simulink model "s9_template"  (R2023a)
settings: Solver=ode4  StartTime=0.0  StopTime=inf  FixedStep=P_sim_dt  RelTol=1e-3
InitFcn:
  | s6_data;
values from neighbouring files (symbols this model uses):
  a1total = 2.7    [mbc_teamchallenge_track.m]    (also in s6_data.m)
  a2total = 1.8    [mbc_teamchallenge_track.m]    (also in s6_data.m)
  breakslen = varargin{1}    [mbc_ppval.m]
  CarInputsCmdForward = uint8(1)    [p_mad_car.m]
  CarInputsCmdHalt = uint8(0)    [p_mad_car.m]
  CarInputsCmdReverse = uint8(2)    [p_mad_car.m]
  ManeuverTypePark = uint8(1)    [p_mad_car.m]
  ManeuverTypePathFollow = uint8(3)    [p_mad_car.m]
  P_cx_k = 1    [s6_data.m]
  P_p_Bf = 0.7    [p_mad_car.m]
  P_p_Br = 0.7    [p_mad_car.m]
  P_p_Cf = 2    [p_mad_car.m]
  P_p_Cr = 2    [p_mad_car.m]
  P_p_delta_max = 21.58/180*pi    (= 0.37664205258)    [p_mad_car.m]
  P_p_Df = 2    [p_mad_car.m]
  P_p_Dr = 2.5    [p_mad_car.m]
  P_p_Ef = -0.1    [p_mad_car.m]
  P_p_Er = -0.05    [p_mad_car.m]
  P_p_J = 192e-6    (= 0.000192)    [p_mad_car.m]
  P_p_k = 2.51    [p_mad_car.m]
  P_p_kr = 0.344014    [s6_data.m]
  P_p_l = abs(P_p_frontaxle_1 + P_p_rearaxle_1)    [p_mad_car.m]
  P_p_lf = P_p_frontaxle_1    (= 0.05)    [p_mad_car.m]
  P_p_lr = P_p_rearaxle_1    (= 0.049)    [p_mad_car.m]
  P_p_m = 132e-3    (= 0.132)    [p_mad_car.m]
  P_p_s1_start = 0.63    [s6_data.m]
  P_p_s2_start = 0.15    [s6_data.m]
  P_p_T = 316e-3    (= 0.316)    [p_mad_car.m]
  P_p_TA = 0.02    [s6_data.m]
  P_p_Ti = 0.246830    (= 0.24683)    [s6_data.m]
  P_p_Tt = P_p_uTt + P_p_output_Tt    (= 0.1)    [p_mad_car.m]
  P_p_Tw = 0.3    [s6_data.m]
  P_w_breakslen = uint32(length(path.points))    [s6_data.m]
  P_w_coefs = zeros(SPLINE.Elements(3).Dimensions)    [s6_data.m]
  P_w_points = zeros(SPLINE.Elements(2).Dimensions)    [s6_data.m]
  P_w_segments = uint32(zeros(SPLINE.Elements(4).Dimensions))    [s6_data.m]
  points = [ p.x + x ;      center1 + sign(t.xe) * r * cos(p.psi - pi/2 + sign(t.xe) * x / t.r) ;      center2 + sign(t.xe) * r * sin(p.psi - pi/2 + sign(t.xe) * x / t.r) ]    [mbc_circle_get_points.m]    (also in mbc_clothoid_get_points.m = [ p.x + x ;      s1;      s2]; mbc_spline_create.m = [ points(:, 1:end-1) [ points(1, end); points(2:3, 1) ] ]; mbc_straight_get_points.m = [ p.x + x ;      p.s1 + cpsi * x + (alpha - 0.5) * t.w * cos)
undefined symbols (not defined in the file or in its folder): coefs, DiscIntNeverNeededParam, periodic, segments
libraries: simulink x1, mad_lib_template x1
settings Model: Creator=hmekiedj  LastModifiedBy=aaron
settings DataIOCC: ReturnWorkspaceOutputs=off
settings OptimizationCC: BlockReduction=off  DefaultParameterBehavior=Inlined  BufferReuse=off
settings DebuggingCC: UnconnectedInputMsg=warning  UnconnectedOutputMsg=warning  UnconnectedLineMsg=warning  ArithmeticOperatorsInVariantConditions=warning
settings ModelReferenceCC: EnableRefExpFcnMdlSchedulingChecks=on
settings SFSimCC: SimUseLocalCustomCode=off  CustomCodeUndefinedFunction=UseInterfaceOnly
settings RTWCC: RTWUseLocalCustomCode=off  DLArmComputeVersion=19.05
settings CodeAppCC: StateflowObjectComments=on

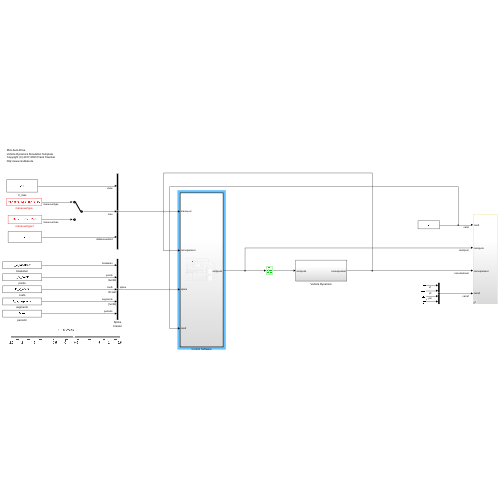
[thumbnail: Simulink's stored preview of the top-level diagram]
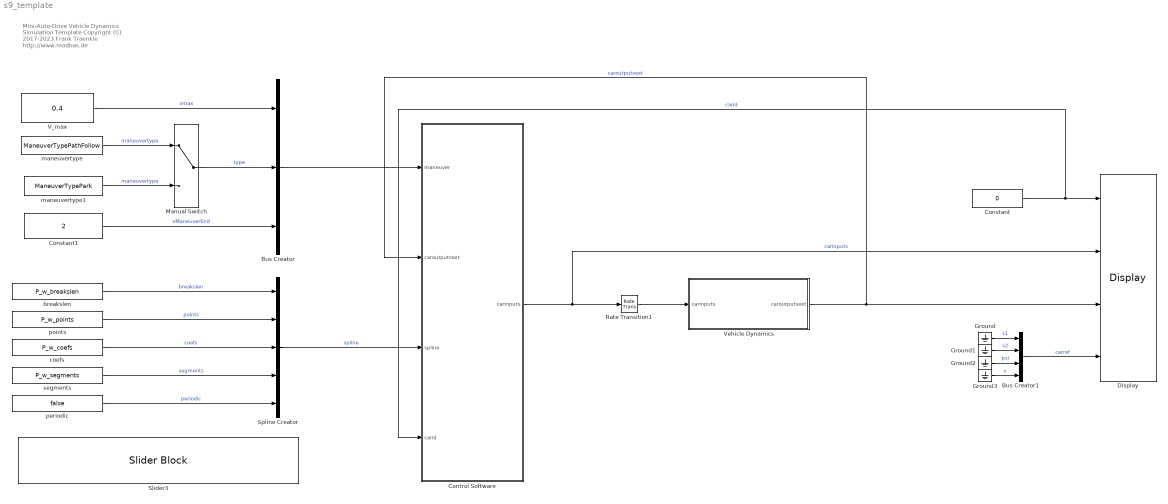
== system s9_template ==
  note: Mini-Auto-Drive
      | Vehicle Dynamics Simulation Template
      | Copyright (C) 2017-2023 Frank Traenkle
      | http://www.modbas.de
  Bus Creator : BusCreator  Inputs=3
  Bus Creator1 : BusCreator  Inputs=4
  Constant : Constant  Value=0
  Constant1 : Constant  Value=2
  Control Software : Subsystem  TreatAsAtomicUnit=on  SystemSampleTime=P_p_TA
  Display : mad_lib_template/Display  SystemSampleTime=-1  VariantActivationTime=update diagram  Latency=0  AutoFrameSizeCalculation=off
  Ground{,1..3} (4 alike) : Ground
  Manual Switch : ManualSwitch
  Rate Transition1 : RateTransition
  Slider3 : SliderBlock  ScaleMin=-2.50  ScaleMax=2.50  TickInterval=0.5
  Spline Creator : BusCreator  Inputs=breakslen,points,coefs,segments,periodic  OutDataTypeStr=Bus: SPLINE
  V_max : Constant  Value=0.4
  Vehicle Dynamics : Subsystem
  breakslen : Constant  Value=P_w_breakslen
  coefs : Constant  Value=P_w_coefs
  maneuvertype : Constant  Value=ManeuverTypePathFollow  SampleTime=-1
  maneuvertype1 : Constant  Value=ManeuverTypePark  SampleTime=-1
  periodic : Constant  Value=false
  points : Constant  Value=P_w_points
  segments : Constant  Value=P_w_segments
  wires:
  Bus Creator1/1 -> Display/4  "carref"
  Ground/1 -> Bus Creator1/1  "s1"
  Ground1/1 -> Bus Creator1/2  "s2"
  Ground2/1 -> Bus Creator1/3  "psi"
  Ground3/1 -> Bus Creator1/4  "v"
  Vehicle Dynamics/1(caroutputsext) -> Control Software/2(caroutputsext), Display/3  "caroutputsext"
  Rate Transition1/1 -> Vehicle Dynamics/1(carinputs)
  Control Software/1(carinputs) -> Display/2, Rate Transition1/1  "carinputs"
  Bus Creator/1 -> Control Software/1(maneuver)
  V_max/1 -> Bus Creator/1  "vmax"
  Manual Switch/1 -> Bus Creator/2  "type"
  maneuvertype/1 -> Manual Switch/1  "maneuvertype"
  maneuvertype1/1 -> Manual Switch/2  "maneuvertype"
  Constant1/1 -> Bus Creator/3  "xManeuverEnd"
  periodic/1 -> Spline Creator/5  "periodic"
  coefs/1 -> Spline Creator/3  "coefs"
  points/1 -> Spline Creator/2  "points"
  breakslen/1 -> Spline Creator/1  "breakslen"
  segments/1 -> Spline Creator/4  "segments"
  Spline Creator/1 -> Control Software/3(spline)  "spline"
  Constant/1 -> Display/1, Control Software/4(carid)  "carid"

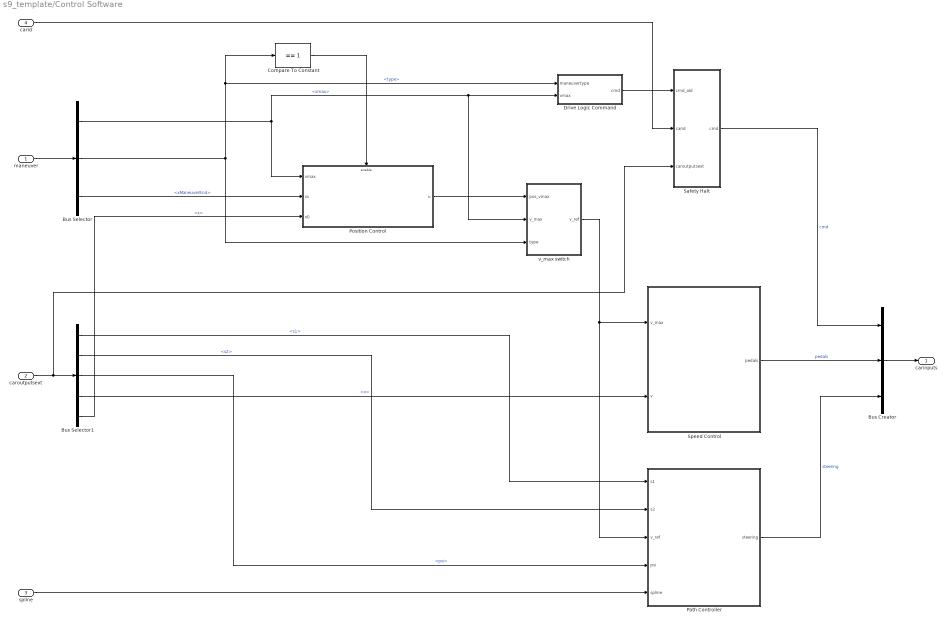
== system s9_template/Control Software ==
  maneuver : Inport
  caroutputsext : Inport  Port=2
  spline : Inport  Port=3
  carid : Inport  Port=4
  Bus Creator : BusCreator  Inputs=3
  Bus Selector : BusSelector  OutputSignals=vmax,type,xManeuverEnd
  Bus Selector1 : BusSelector  OutputSignals=s1,s2,psi,v,x
  Compare To Constant : simulink/Logic and Bit Operations/Compare To Constant  relop===  const=1  OutDataTypeStr=boolean
  Drive Logic Command : MATLAB Function  TreatAsAtomicUnit=on
  Path Controller : Subsystem
  Position Control : Subsystem  TreatAsAtomicUnit=on
  Safety Halt : MATLAB Function  TreatAsAtomicUnit=on
  Speed Control : Subsystem
  v_max switch : MATLAB Function  TreatAsAtomicUnit=on
  carinputs : Outport
  wires:
  caroutputsext/1 -> Bus Selector1/1, Safety Halt/3(caroutputsext)
  Position Control/1(u) -> v_max switch/1(pos_vmax)
  maneuver/1 -> Bus Selector/1
  Bus Selector/1 -> Position Control/1(vmax), v_max switch/2(v_max), Drive Logic Command/2(vmax)  "<vmax>"
  Bus Selector1/5 -> Position Control/3(x0)  "<x>"
  Bus Selector/2 -> v_max switch/3(type), Compare To Constant/1, Drive Logic Command/1(maneuvertype)  "<type>"
  Compare To Constant/1 -> Position Control/Enable
  Bus Creator/1 -> carinputs/1
  Bus Selector/3 -> Position Control/2(xs)  "<xManeuverEnd>"
  Bus Selector1/1 -> Path Controller/1(s1)  "<s1>"
  Bus Selector1/2 -> Path Controller/2(s2)  "<s2>"
  Bus Selector1/3 -> Path Controller/4(psi)  "<psi>"
  v_max switch/1(v_ref) -> Path Controller/3(v_ref), Speed Control/1(v_max)
  Drive Logic Command/1(cmd) -> Safety Halt/1(cmd_old)
  Path Controller/1(steering) -> Bus Creator/3  "steering"
  spline/1 -> Path Controller/5(spline)
  Bus Selector1/4 -> Speed Control/2(v)  "<v>"
  Speed Control/1(pedals) -> Bus Creator/2  "pedals"
  Safety Halt/1(cmd) -> Bus Creator/1  "cmd"
  carid/1 -> Safety Halt/2(carid)

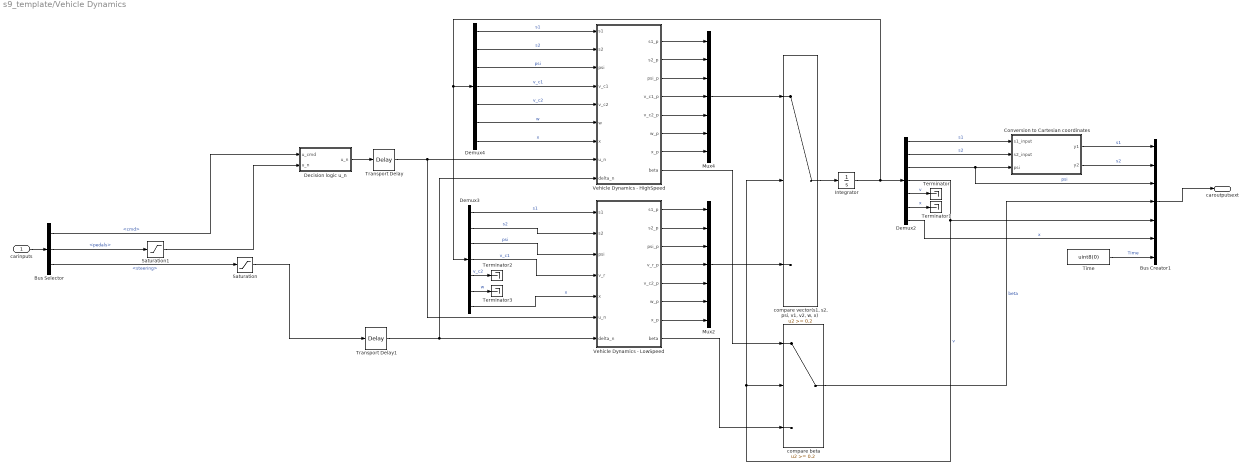
== system s9_template/Vehicle Dynamics ==
  carinputs : Inport
  Bus Creator1 : BusCreator  Inputs=7  OutDataTypeStr=Bus: CAROUTPUTSEXT
  Bus Selector : BusSelector  OutputSignals=cmd,pedals,steering
  Conversion to Cartesian coordinates : MATLAB Function  TreatAsAtomicUnit=on
  Decision logic u_n : MATLAB Function  TreatAsAtomicUnit=on
  Demux2 : Demux  Outputs=7
  Demux3 : Demux  Outputs=7
  Demux4 : Demux  Outputs=7
  Integrator : Integrator  InitialCondition=[P_p_s1_start; P_p_s2_start; 0; 0; 0; 0; 0]
  Mux2 : Mux  Inputs=7
  Mux4 : Mux  Inputs=7
  Saturation : Saturate  UpperLimit=1  LowerLimit=-1
  Saturation1 : Saturate  UpperLimit=1  LowerLimit=-1
  Terminator{,1..3} (4 alike) : Terminator
  Time : Constant  Value=uint8(0)
  Transport Delay : TransportDelay  DelayTime=P_p_Tt
  Transport Delay1 : TransportDelay  DelayTime=P_p_Tt
  Vehicle Dynamics - HighSpeed : Subsystem
  Vehicle Dynamics - LowSpeed : Subsystem
  compare beta : Switch  Threshold=0.2  SaturateOnIntegerOverflow=off  InputSameDT=off
  "compare vector(s1, s2, psi, v1, v2, w, x)" : Switch  Threshold=0.2  SaturateOnIntegerOverflow=off  InputSameDT=off
  caroutputsext : Outport  VectorParamsAs1DForOutWhenUnconnected=off
  wires:
  carinputs/1 -> Bus Selector/1
  Bus Selector/2 -> Saturation1/1  "<pedals>"
  Bus Selector/3 -> Saturation/1  "<steering>"
  Demux2/3 -> Conversion to Cartesian coordinates/3(psi), Bus Creator1/3  "psi"
  Bus Creator1/1 -> caroutputsext/1
  Demux2/7 -> Bus Creator1/6  "x"
  Demux2/2 -> Conversion to Cartesian coordinates/2(s2_input)  "s2"
  Demux2/1 -> Conversion to Cartesian coordinates/1(s1_input)  "s1"
  Bus Selector/1 -> Decision logic u_n/1(u_cmd)  "<cmd>"
  Saturation1/1 -> Decision logic u_n/2("u_n ")
  Saturation/1 -> Transport Delay1/1
  Vehicle Dynamics - HighSpeed/1(s1_p) -> Mux4/1
  Vehicle Dynamics - HighSpeed/2(s2_p) -> Mux4/2
  Vehicle Dynamics - HighSpeed/3(psi_p) -> Mux4/3
  Vehicle Dynamics - HighSpeed/4(v_c1_p) -> Mux4/4
  Vehicle Dynamics - HighSpeed/5(v_c2_p) -> Mux4/5
  Vehicle Dynamics - HighSpeed/6(w_p) -> Mux4/6
  Vehicle Dynamics - HighSpeed/7(x_p) -> Mux4/7
  Vehicle Dynamics - LowSpeed/1(s1_p) -> Mux2/1
  Vehicle Dynamics - LowSpeed/2(s2_p) -> Mux2/2
  Vehicle Dynamics - LowSpeed/3(psi_p) -> Mux2/3
  Vehicle Dynamics - LowSpeed/4(v_r_p) -> Mux2/4
  Vehicle Dynamics - LowSpeed/5(v_c2_p) -> Mux2/5
  Vehicle Dynamics - LowSpeed/6(w_p) -> Mux2/6
  Vehicle Dynamics - LowSpeed/7(x_p) -> Mux2/7
  Mux4/1 -> "compare vector(s1, s2, psi, v1, v2, w, x)"/1
  "compare vector(s1, s2, psi, v1, v2, w, x)"/1 -> Integrator/1
  Integrator/1 -> Demux2/1, Demux4/1, Demux3/1
  Demux2/4 -> "compare vector(s1, s2, psi, v1, v2, w, x)"/2, compare beta/2, Bus Creator1/5  "v"
  Demux3/1 -> Vehicle Dynamics - LowSpeed/1(s1)  "s1"
  Demux3/2 -> Vehicle Dynamics - LowSpeed/2(s2)  "s2"
  Demux3/3 -> Vehicle Dynamics - LowSpeed/3(psi)  "psi"
  Demux3/4 -> Vehicle Dynamics - LowSpeed/4(v_r)  "v_c1"
  Demux3/7 -> Vehicle Dynamics - LowSpeed/5(x)  "x"
  Demux4/1 -> Vehicle Dynamics - HighSpeed/1(s1)  "s1"
  Demux4/2 -> Vehicle Dynamics - HighSpeed/2(s2)  "s2"
  Demux4/3 -> Vehicle Dynamics - HighSpeed/3(psi)  "psi"
  Demux4/4 -> Vehicle Dynamics - HighSpeed/4(v_c1)  "v_c1"
  Demux4/5 -> Vehicle Dynamics - HighSpeed/5(v_c2)  "v_c2"
  Demux4/6 -> Vehicle Dynamics - HighSpeed/6(w)  "w"
  Demux4/7 -> Vehicle Dynamics - HighSpeed/7(x)  "x"
  Transport Delay/1 -> Vehicle Dynamics - LowSpeed/6(u_n), Vehicle Dynamics - HighSpeed/8(u_n)
  Transport Delay1/1 -> Vehicle Dynamics - LowSpeed/7(delta_n), Vehicle Dynamics - HighSpeed/9(delta_n)
  Vehicle Dynamics - LowSpeed/8(beta) -> compare beta/3
  Vehicle Dynamics - HighSpeed/8(beta) -> compare beta/1
  compare beta/1 -> Bus Creator1/4  "beta"
  Conversion to Cartesian coordinates/1(y1) -> Bus Creator1/1  "s1"
  Conversion to Cartesian coordinates/2(y2) -> Bus Creator1/2  "s2"
  Demux2/5 -> Terminator/1  "v"
  Demux2/6 -> Terminator1/1  "x"
  Decision logic u_n/1(u_n) -> Transport Delay/1
  Demux3/5 -> Terminator2/1  "v_c2"
  Demux3/6 -> Terminator3/1  "w"
  Mux2/1 -> "compare vector(s1, s2, psi, v1, v2, w, x)"/3
  Time/1 -> Bus Creator1/7  "Time"

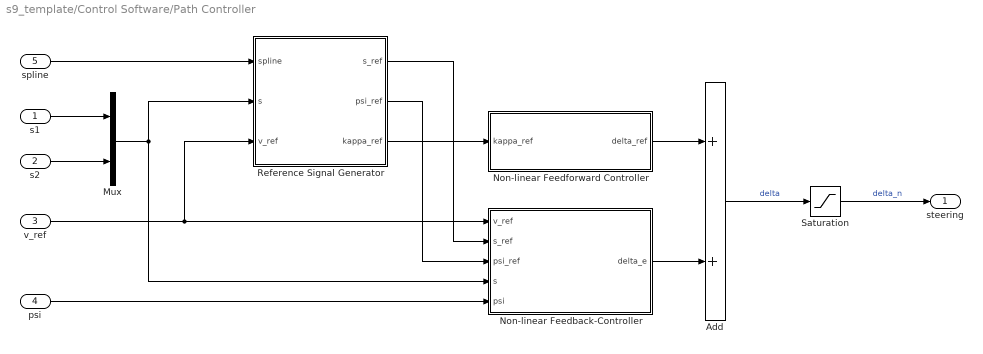
== system s9_template/Control Software/Path Controller ==
  s1 : Inport
  s2 : Inport  Port=2
  v_ref : Inport  Port=3
  psi : Inport  Port=4
  spline : Inport  Port=5
  Add : Sum
  Mux : Mux  Inputs=2
  Non-linear Feedback-Controller : MATLAB Function  TreatAsAtomicUnit=on
  Non-linear Feedforward Controller : MATLAB Function  TreatAsAtomicUnit=on
  Reference Signal Generator : MATLAB Function  TreatAsAtomicUnit=on
  Saturation : Saturate  UpperLimit=1  LowerLimit=-1
  steering : Outport
  wires:
  spline/1 -> Reference Signal Generator/1(spline)
  s1/1 -> Mux/1
  s2/1 -> Mux/2
  v_ref/1 -> Reference Signal Generator/3(v_ref), Non-linear Feedback-Controller/1(v_ref)
  Reference Signal Generator/3(kappa_ref) -> Non-linear Feedforward Controller/1(kappa_ref)
  Reference Signal Generator/2(psi_ref) -> Non-linear Feedback-Controller/3(psi_ref)
  Reference Signal Generator/1(s_ref) -> Non-linear Feedback-Controller/2(s_ref)
  Non-linear Feedforward Controller/1(delta_ref) -> Add/1
  Non-linear Feedback-Controller/1(delta_e) -> Add/2
  Add/1 -> Saturation/1  "delta"
  Saturation/1 -> steering/1  "delta_n"
  Mux/1 -> Reference Signal Generator/2(s), Non-linear Feedback-Controller/4(s)
  psi/1 -> Non-linear Feedback-Controller/5(psi)

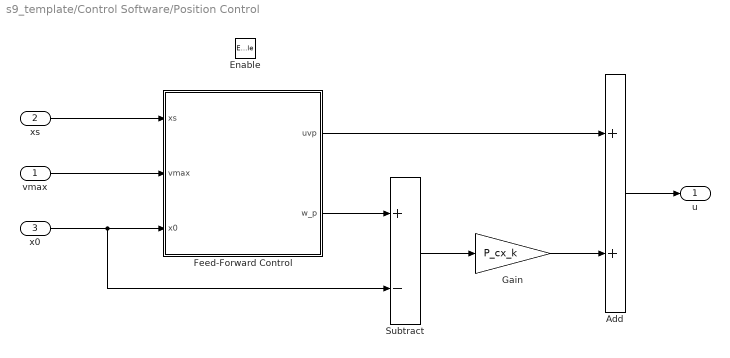
== system s9_template/Control Software/Position Control ==
  vmax : Inport
  xs : Inport  Port=2
  x0 : Inport  Port=3
  Enable : EnablePort
  Add : Sum
  Feed-Forward Control : Subsystem
  Gain : Gain  Gain=P_cx_k
  Subtract : Sum  Inputs=+-
  u : Outport
  wires:
  xs/1 -> Feed-Forward Control/1(xs)
  Feed-Forward Control/2(w_p) -> Subtract/1
  Subtract/1 -> Gain/1
  Feed-Forward Control/1(uvp) -> Add/1
  vmax/1 -> Feed-Forward Control/2(vmax)
  Gain/1 -> Add/2
  Add/1 -> u/1
  x0/1 -> Subtract/2, Feed-Forward Control/3(x0)

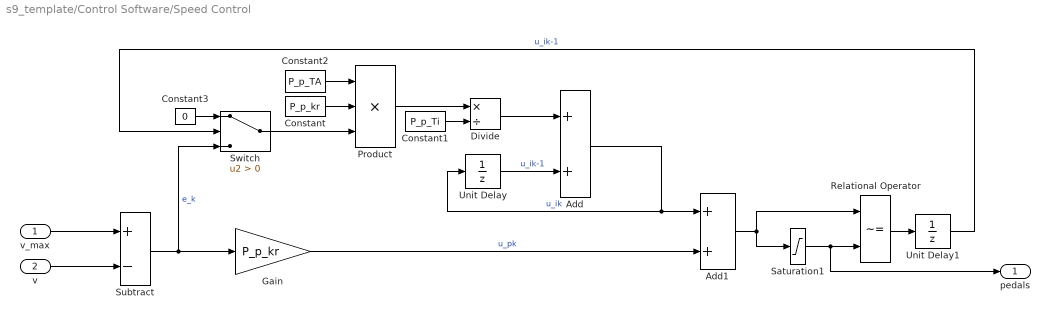
== system s9_template/Control Software/Speed Control ==
  v_max : Inport
  v : Inport  Port=2
  Add : Sum
  Add1 : Sum
  Constant : Constant  Value=P_p_kr
  Constant1 : Constant  Value=P_p_Ti  VectorParams1D=off
  Constant2 : Constant  Value=P_p_TA  VectorParams1D=off
  Constant3 : Constant  Value=0
  Divide : Product  Inputs=*/
  Gain : Gain  Gain=P_p_kr
  Product : Product  Inputs=3
  Relational Operator : RelationalOperator  Operator=~=  OutDataTypeStr=boolean  RndMeth=Simplest  InputSameDT=off
  Saturation1 : Saturate  UpperLimit=1  LowerLimit=-1
  Subtract : Sum  Inputs=+-
  Switch : Switch  Criteria=u2 > Threshold  SaturateOnIntegerOverflow=off  InputSameDT=off
  Unit Delay : UnitDelay  SampleTime=P_p_TA  HasFrameUpgradeWarning=on
  Unit Delay1 : UnitDelay  SampleTime=P_p_TA  HasFrameUpgradeWarning=on
  pedals : Outport
  wires:
  Constant3/1 -> Switch/1
  Relational Operator/1 -> Unit Delay1/1
  Divide/1 -> Add/1
  Subtract/1 -> Gain/1, Switch/3  "e_k"
  Constant2/1 -> Product/1
  Saturation1/1 -> Relational Operator/2, pedals/1
  Switch/1 -> Product/3
  Constant/1 -> Product/2
  Constant1/1 -> Divide/2
  Product/1 -> Divide/1
  Unit Delay1/1 -> Switch/2  "u_ik-1"
  Gain/1 -> Add1/2  "u_pk"
  Unit Delay/1 -> Add/2  "u_ik-1"
  Add/1 -> Add1/1, Unit Delay/1  "u_ik"
  Add1/1 -> Relational Operator/1, Saturation1/1
  v_max/1 -> Subtract/1
  v/1 -> Subtract/2

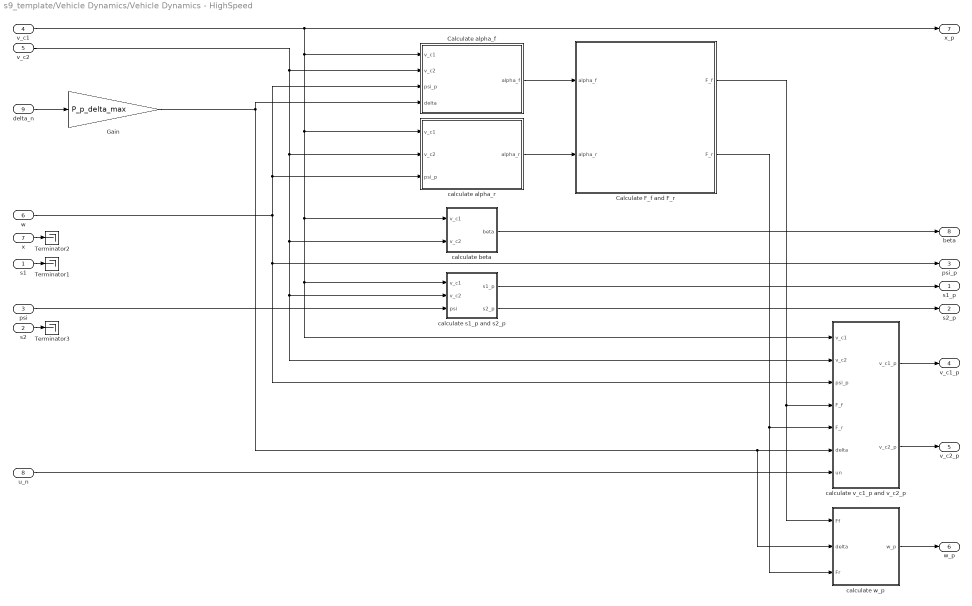
== system s9_template/Vehicle Dynamics/Vehicle Dynamics - HighSpeed ==
  s1 : Inport
  s2 : Inport  Port=2
  psi : Inport  Port=3
  v_c1 : Inport  Port=4
  v_c2 : Inport  Port=5
  w : Inport  Port=6
  x : Inport  Port=7
  u_n : Inport  Port=8
  delta_n : Inport  Port=9
  Calculate F_f and F_r : MATLAB Function  TreatAsAtomicUnit=on
  Calculate alpha_f : MATLAB Function  TreatAsAtomicUnit=on
  Gain : Gain  Gain=P_p_delta_max
  Terminator1 : Terminator
  Terminator2 : Terminator
  Terminator3 : Terminator
  calculate alpha_r : MATLAB Function  TreatAsAtomicUnit=on
  calculate beta : MATLAB Function  TreatAsAtomicUnit=on
  calculate s1_p and s2_p : MATLAB Function  TreatAsAtomicUnit=on
  calculate v_c1_p and v_c2_p : MATLAB Function  TreatAsAtomicUnit=on
  calculate w_p : MATLAB Function  TreatAsAtomicUnit=on
  s1_p : Outport  VectorParamsAs1DForOutWhenUnconnected=off
  s2_p : Outport  Port=2  VectorParamsAs1DForOutWhenUnconnected=off
  psi_p : Outport  Port=3  VectorParamsAs1DForOutWhenUnconnected=off
  v_c1_p : Outport  Port=4  VectorParamsAs1DForOutWhenUnconnected=off
  v_c2_p : Outport  Port=5  VectorParamsAs1DForOutWhenUnconnected=off
  w_p : Outport  Port=6  VectorParamsAs1DForOutWhenUnconnected=off
  x_p : Outport  Port=7  VectorParamsAs1DForOutWhenUnconnected=off
  beta : Outport  Port=8  VectorParamsAs1DForOutWhenUnconnected=off
  wires:
  delta_n/1 -> Gain/1
  Calculate alpha_f/1(alpha_f) -> Calculate F_f and F_r/1(alpha_f)
  calculate alpha_r/1(alpha_r) -> Calculate F_f and F_r/2(alpha_r)
  calculate beta/1(beta) -> beta/1
  calculate s1_p and s2_p/1(s1_p) -> s1_p/1
  calculate s1_p and s2_p/2(s2_p) -> s2_p/1
  Gain/1 -> calculate v_c1_p and v_c2_p/6(delta), calculate w_p/2(delta), Calculate alpha_f/4(delta)
  w/1 -> psi_p/1, calculate v_c1_p and v_c2_p/3(psi_p), calculate alpha_r/3(psi_p), Calculate alpha_f/3(psi_p)
  u_n/1 -> calculate v_c1_p and v_c2_p/7(un)
  Calculate F_f and F_r/2(F_r) -> calculate w_p/3(Fr), calculate v_c1_p and v_c2_p/5(F_r)
  Calculate F_f and F_r/1(F_f) -> calculate w_p/1(Ff), calculate v_c1_p and v_c2_p/4(F_f)
  calculate v_c1_p and v_c2_p/1(v_c1_p) -> v_c1_p/1
  calculate v_c1_p and v_c2_p/2(v_c2_p) -> v_c2_p/1
  v_c1/1 -> calculate v_c1_p and v_c2_p/1(v_c1), calculate s1_p and s2_p/1(v_c1), calculate beta/1(v_c1), calculate alpha_r/1(v_c1), Calculate alpha_f/1(v_c1), x_p/1
  v_c2/1 -> calculate v_c1_p and v_c2_p/2(v_c2), calculate s1_p and s2_p/2(v_c2), calculate beta/2(v_c2), calculate alpha_r/2(v_c2), Calculate alpha_f/2(v_c2)
  calculate w_p/1(w_p) -> w_p/1
  psi/1 -> calculate s1_p and s2_p/3(psi)
  x/1 -> Terminator2/1
  s1/1 -> Terminator1/1
  s2/1 -> Terminator3/1

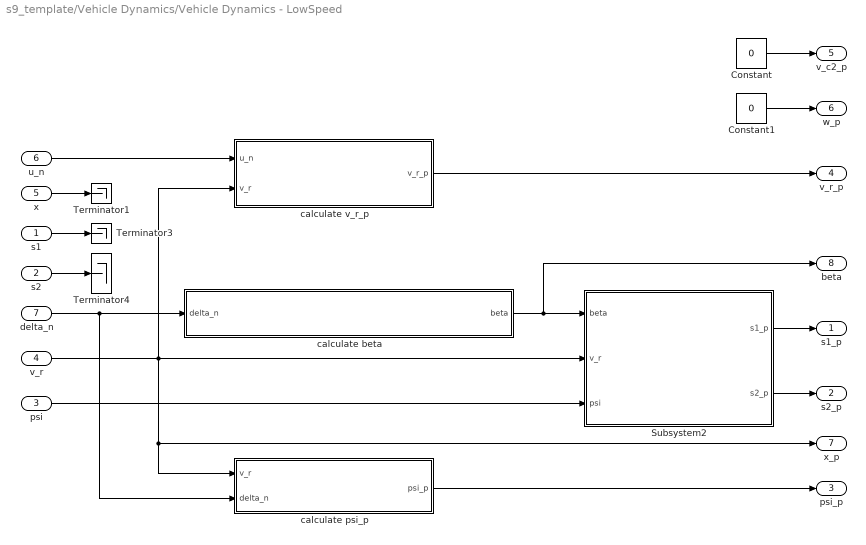
== system s9_template/Vehicle Dynamics/Vehicle Dynamics - LowSpeed ==
  s1 : Inport
  s2 : Inport  Port=2
  psi : Inport  Port=3
  v_r : Inport  Port=4
  x : Inport  Port=5
  u_n : Inport  Port=6
  delta_n : Inport  Port=7
  Constant : Constant  Value=0
  Constant1 : Constant  Value=0
  Subsystem2 : Subsystem
  Terminator1 : Terminator
  Terminator3 : Terminator
  Terminator4 : Terminator
  calculate beta : Subsystem
  calculate psi_p : Subsystem
  calculate v_r_p : Subsystem
  s1_p : Outport  VectorParamsAs1DForOutWhenUnconnected=off
  s2_p : Outport  Port=2  VectorParamsAs1DForOutWhenUnconnected=off
  psi_p : Outport  Port=3  VectorParamsAs1DForOutWhenUnconnected=off
  v_r_p : Outport  Port=4  VectorParamsAs1DForOutWhenUnconnected=off
  v_c2_p : Outport  Port=5  VectorParamsAs1DForOutWhenUnconnected=off
  w_p : Outport  Port=6  VectorParamsAs1DForOutWhenUnconnected=off
  x_p : Outport  Port=7  VectorParamsAs1DForOutWhenUnconnected=off
  beta : Outport  Port=8  VectorParamsAs1DForOutWhenUnconnected=off
  wires:
  u_n/1 -> calculate v_r_p/1(u_n)
  calculate v_r_p/1(v_r_p) -> v_r_p/1
  v_r/1 -> calculate psi_p/1(v_r), x_p/1, Subsystem2/2(v_r), calculate v_r_p/2(v_r)
  delta_n/1 -> calculate psi_p/2(delta_n), calculate beta/1(delta_n)
  Subsystem2/1(s1_p) -> s1_p/1
  psi/1 -> Subsystem2/3(psi)
  calculate beta/1(beta) -> Subsystem2/1(beta), beta/1
  Subsystem2/2(s2_p) -> s2_p/1
  calculate psi_p/1(psi_p) -> psi_p/1
  x/1 -> Terminator1/1
  s1/1 -> Terminator3/1
  s2/1 -> Terminator4/1
  Constant/1 -> v_c2_p/1
  Constant1/1 -> w_p/1

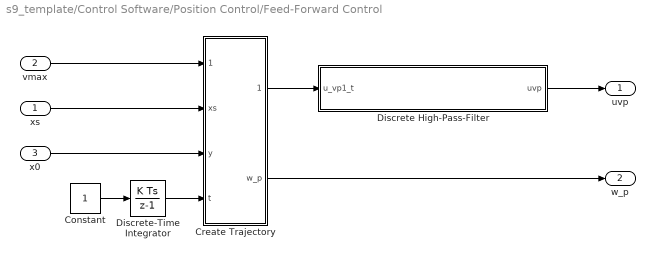
== system s9_template/Control Software/Position Control/Feed-Forward Control ==
  xs : Inport
  vmax : Inport  Port=2
  x0 : Inport  Port=3
  Constant : Constant
  "Create Trajectory " : MATLAB Function  TreatAsAtomicUnit=on
  Discrete High-Pass-Filter : Subsystem  TreatAsAtomicUnit=on
  Discrete-Time Integrator : DiscreteIntegrator  SampleTime=-1  ICPrevOutput=DiscIntNeverNeededParam  ICPrevScaledInput=DiscIntNeverNeededParam
  uvp : Outport
  w_p : Outport  Port=2
  wires:
  x0/1 -> "Create Trajectory "/3(y)
  vmax/1 -> "Create Trajectory "/1(vmax)
  xs/1 -> "Create Trajectory "/2(xs)
  "Create Trajectory "/2(w_p) -> w_p/1
  "Create Trajectory "/1(u_vp1_t) -> Discrete High-Pass-Filter/1(u_vp1_t)
  Constant/1 -> Discrete-Time Integrator/1
  Discrete-Time Integrator/1 -> "Create Trajectory "/4(t)
  Discrete High-Pass-Filter/1(uvp) -> uvp/1

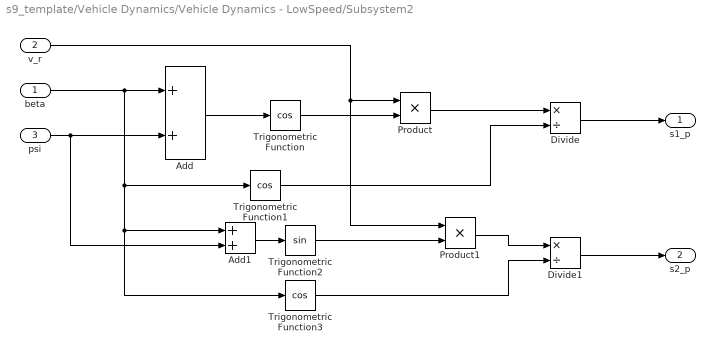
== system s9_template/Vehicle Dynamics/Vehicle Dynamics - LowSpeed/Subsystem2 ==
  beta : Inport
  v_r : Inport  Port=2
  psi : Inport  Port=3
  Add : Sum
  Add1 : Sum
  Divide : Product  Inputs=*/
  Divide1 : Product  Inputs=*/
  Product : Product
  Product1 : Product
  Trigonometric Function : Trigonometry  Operator=cos
  Trigonometric Function1 : Trigonometry  Operator=cos
  Trigonometric Function2 : Trigonometry
  Trigonometric Function3 : Trigonometry  Operator=cos
  s1_p : Outport  VectorParamsAs1DForOutWhenUnconnected=off
  s2_p : Outport  Port=2  VectorParamsAs1DForOutWhenUnconnected=off
  wires:
  Add/1 -> Trigonometric Function/1
  Trigonometric Function/1 -> Product/2
  Product/1 -> Divide/1
  Trigonometric Function1/1 -> Divide/2
  Divide/1 -> s1_p/1
  psi/1 -> Add1/2, Add/2
  beta/1 -> Trigonometric Function1/1, Trigonometric Function3/1, Add1/1, Add/1
  Trigonometric Function2/1 -> Product1/2
  Divide1/1 -> s2_p/1
  v_r/1 -> Product1/1, Product/1
  Product1/1 -> Divide1/1
  Add1/1 -> Trigonometric Function2/1
  Trigonometric Function3/1 -> Divide1/2

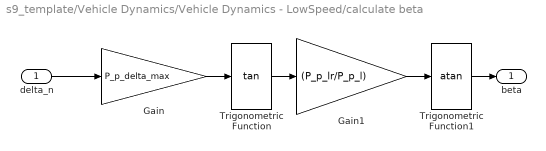
== system s9_template/Vehicle Dynamics/Vehicle Dynamics - LowSpeed/calculate beta ==
  delta_n : Inport
  Gain : Gain  Gain=P_p_delta_max
  Gain1 : Gain  Gain=(P_p_lr/P_p_l)
  Trigonometric Function : Trigonometry  Operator=tan
  Trigonometric Function1 : Trigonometry  Operator=atan
  beta : Outport  VectorParamsAs1DForOutWhenUnconnected=off
  wires:
  delta_n/1 -> Gain/1
  Gain/1 -> Trigonometric Function/1
  Trigonometric Function/1 -> Gain1/1
  Gain1/1 -> Trigonometric Function1/1
  Trigonometric Function1/1 -> beta/1

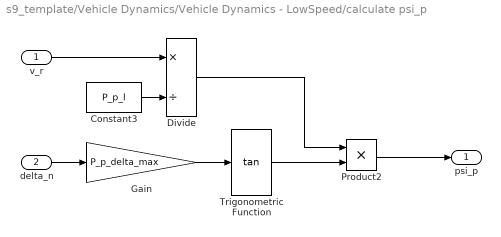
== system s9_template/Vehicle Dynamics/Vehicle Dynamics - LowSpeed/calculate psi_p ==
  v_r : Inport
  delta_n : Inport  Port=2
  Constant3 : Constant  Value=P_p_l
  Divide : Product  Inputs=*/
  Gain : Gain  Gain=P_p_delta_max
  Product2 : Product
  Trigonometric Function : Trigonometry  Operator=tan
  psi_p : Outport  VectorParamsAs1DForOutWhenUnconnected=off
  wires:
  delta_n/1 -> Gain/1
  Gain/1 -> Trigonometric Function/1
  Product2/1 -> psi_p/1
  v_r/1 -> Divide/1
  Constant3/1 -> Divide/2
  Trigonometric Function/1 -> Product2/2
  Divide/1 -> Product2/1

== system s9_template/Vehicle Dynamics/Vehicle Dynamics - LowSpeed/calculate v_r_p ==
  u_n : Inport
  v_r : Inport  Port=2
  Add : Sum  Inputs=-+
  Gain : Gain  Gain=(1/P_p_T)
  Gain1 : Gain  Gain=(P_p_k/P_p_T)
  v_r_p : Outport  VectorParamsAs1DForOutWhenUnconnected=off
  wires:
  Gain/1 -> Add/1
  Add/1 -> v_r_p/1
  v_r/1 -> Gain/1
  u_n/1 -> Gain1/1
  Gain1/1 -> Add/2

== system s9_template/Control Software/Position Control/Feed-Forward Control/Discrete High-Pass-Filter ==
  u_vp1_t : Inport
  Discrete High-Pass-Filter : DiscreteTransferFcn  Numerator=[2, -2]  Denominator=[(2*P_p_Ti+P_p_T) (P_p_T-2*P_p_Ti)]
  uvp : Outport
  wires:
  Discrete High-Pass-Filter/1 -> uvp/1
  u_vp1_t/1 -> Discrete High-Pass-Filter/1

== matlab function s9_template/Vehicle Dynamics/Vehicle Dynamics - HighSpeed/calculate v_c1_p and v_c2_p ==
  data: v_c1 input; v_c1_p output; v_c2 input; psi_p input; v_c2_p output; F_f input; F_r input; delta input; un input; P_p_m parameter; P_p_T parameter; P_p_k parameter
function [v_c1_p, v_c2_p] = fcn(v_c1, v_c2, psi_p, F_f, F_r, delta, un, P_p_m, P_p_T, P_p_k)
    % Function: fcn
    % Description: Calculates the updated longitudinal and lateral velocity components 
    %              of a vehicle based on various dynamic parameters and forces.
    %
    % Inputs:
    %   v_c1 - Initial longitudinal velocity component.
    %   v_c2 - Initial lateral velocity component.
    %   psi_p - Yaw rate of the vehicle.
    %   F_f - Tire force at the front of the vehicle.
    %   F_r - Tire force at the rear of the vehicle.
    %   delta - Steering angle.
    %   un - Motor control signal.
    %   P_p_m - Mass of the vehicle.
    %   P_p_T - Time constant related to the vehicle dynamics.
    %   P_p_k - Constant related to the motor control effectiveness.
    %
    % Outputs:
    %   v_c1_p - Updated longitudinal velocity component.
    %   v_c2_p - Updated lateral velocity component.
    %
    % The function calculates the new velocity components considering the external forces,
    % vehicle's yaw rate, steering angle, motor control signal, and various vehicle parameters.
    % These calculations are essential for understanding the vehicle's dynamic behavior under
    % different control inputs and conditions.
    
    % Calculating the updated velocity components
    v_c1_p = double((1 / P_p_m) * (-F_f * sin(delta) + (P_p_m * v_c2 * psi_p)) - (1 / P_p_T * v_c1) + ((P_p_k / P_p_T) * un));
    v_c2_p = double((1 / P_p_m) * (F_f * cos(delta) + F_r - (P_p_m * v_c1 * psi_p)));
end

== matlab function s9_template/Vehicle Dynamics/Vehicle Dynamics - HighSpeed/calculate w_p ==
  data: w_p output; Ff input; delta input; Fr input; P_p_J parameter; P_p_lf parameter; P_p_lr parameter
function w_p = fcn(Ff, delta, Fr, P_p_J, P_p_lf, P_p_lr)
    % Function: fcn
    % Description: Calculates the yaw rate change 'w_p' of a vehicle.
    %
    % Inputs:
    %   Ff - Front tire force.
    %   delta - Steering angle.
    %   Fr - Rear tire force.
    %   P_p_J - Moment of inertia of the vehicle about the yaw axis.
    %   P_p_lf - Distance from the center of gravity (COG) to the front axle.
    %   P_p_lr - Distance from the COG to the rear axle.
    %
    % Output:
    %   w_p - Calculated change in yaw rate.
    %
    % The function computes the change in the vehicle's yaw rate based on the forces 
    % acting on the front and rear tires, the steering angle, the vehicle's moment of 
    % inertia, and the distances from the COG to the front and rear axles. This calculation 
    % is crucial for understanding the vehicle's dynamic response to steering inputs.
    
    % Calculation of the yaw rate change 'w_p'
    w_p = 1 / P_p_J * (Ff * P_p_lf * cos(delta) - Fr * P_p_lr);
end

== matlab function s9_template/Control Software/Drive Logic Command ==
  data: maneuvertype input; vmax input; cmd output
function cmd = fcn(maneuvertype, vmax)
    % Function: fcn
    % Description: Determines the appropriate command for vehicle maneuver based on the 
    %              maneuver type and maximum velocity.
    %
    % Inputs:
    %   maneuvertype - Numeric value indicating the type of maneuver.
    %   vmax - Maximum velocity 
    %   CarInputsCmdReverse - Command for reversing the vehicle.
    %   CarInputsCmdForward - Command for moving the vehicle forward.
    %   CarInputsCmdSlow - Command for slowing down the vehicle.
    %
    % Output:
    %   cmd - The calculated command for the vehicle maneuver.
    %
    % The function sets the command for a vehicle maneuver based on the maneuver type and 
    % maximum velocity. If the maneuver type is 1, it sets the command to slow down. Otherwise, 
    % it chooses between moving forward or reversing based on the maximum velocity.

    % Setting the initial command to forward    
    % Logic to determine the command based on maneuver type and maximum velocity
    % if maneuvertype == 1
    %     cmd = CarInputsCmdSlow;
    % else
    %     if vmax >= 0
    %         cmd = CarInputsCmdForward;
    %     elseif vmax < 0
    %         cmd = CarInputsCmdReverse;
    %     end 
    % end
    cmd = 1;   % "CarInputsCmdForward"
      switch maneuvertype
        case 0      % CarInputsCmdHalt
            cmd = 0;
        case 1  % CarInputsCmdForward 
            if (vmax < 0)
                cmd = 0;
            end
        case 2  % CarInputsCmdReverse 
            if (vmax > 0)
                cmd = 0;
            end
     end
end

== matlab function s9_template/Control Software/Path Controller/Reference Signal Generator ==
  data: spline input; s_ref output; s input size=2; v_ref input size=1; psi_ref output; kappa_ref output; P_p_Tt parameter
function [s_ref, psi_ref, kappa_ref] = E_ref(spline, s, v_ref, P_p_Tt)
    % Function: E_ref
    % Description: Calculates reference values for position, orientation, and curvature
    %              based on a given spline, position, and velocity.
    %
    % Inputs:
    %   spline - Spline structure containing points, coefficients, lengths, and periodicity.
    %   s - Current position along the spline.
    %   v_ref - Reference velocity.
    %   P_p_Tt - Dead time affecting the response.
    %
    % Outputs:
    %   s_ref - Reference position in terms of x and y coordinates.
    %   psi_ref - Reference orientation (yaw angle).
    %   kappa_ref - Reference curvature.
    %
    % The function uses the spline data along with the current position and reference velocity
    % to determine the reference position (s_ref), orientation (psi_ref), and curvature (kappa_ref).
    % These are crucial for path following and trajectory planning in vehicle dynamics.
    %

    % Extracting spline components
    points = spline.points;
    coefs = spline.coefs;
    breakslen = spline.breakslen;
    periodic = spline.periodic;
    
    % Calculating reference values using spline data
    [w, widx] = mbc_spline_get_reference(s, breakslen, points, coefs, periodic, v_ref, P_p_Tt);
    
    % Assigning the calculated reference values
    psi_ref = w(2);
    kappa_ref = w(5);
    s_ref = [w(3), w(4)];
end

== matlab function s9_template/Control Software/Path Controller/Non-linear Feedforward Controller ==
  data: kappa_ref input; delta_ref output; P_p_l parameter
function delta_ref = E_FF(kappa_ref, P_p_l)
    % Function: E_FF
    % Description: Calculates the reference steering angle 'delta_ref' for feedforward control.
    %
    % Inputs:
    %   kappa_ref - Reference curvature of the path.
    %   P_p_l - Wheelbase length of the vehicle.
    %
    % Output:
    %   delta_ref - Calculated reference steering angle for feedforward control.
    %
    % The function computes the reference steering angle (delta_ref) needed for a vehicle
    % to follow a path with a given curvature (kappa_ref). This calculation is crucial in
    % feedforward control systems where precise steering based on the path's curvature is required.
    %

    % Calculating the reference steering angle based on the curvature and wheelbase
    delta_ref = atan(P_p_l * kappa_ref);
end

== matlab function s9_template/Control Software/Path Controller/Non-linear Feedback-Controller ==
  data: v_ref input; delta_e output; s_ref input; psi_ref input; s input; psi input; P_p_Tw parameter; P_p_l parameter
function delta_e = E_FB(v_ref, s_ref, psi_ref, s, psi, P_p_Tw, P_p_l)
    % Function: E_FB
    % Description: Calculates the steering angle error 'delta_e' for feedback control in vehicle dynamics.
    %
    % Inputs:
    %   v_ref - Reference velocity.
    %   s_ref - Reference position coordinates (x_ref, y_ref).
    %   psi_ref - Reference orientation (yaw angle).
    %   s - Current position coordinates (x, y).
    %   psi - Current orientation (yaw angle).
    %   P_p_Tw - Time constant Tw.
    %   P_p_l - Wheelbase length of the vehicle.
    %
    % Output:
    %   delta_e - Calculated error in steering angle.
    %
    % The function computes the error in the steering angle for feedback control. It first
    % normalizes the orientation error and calculates the lateral position error. The function
    % then adjusts the reference velocity if it's within a certain range for accuracy. Finally,
    % it uses these errors to calculate the steering angle error based on the vehicle's dynamics.

    % Calculate orientation error and normalize
    psi_e = psi - psi_ref;
    psi_e = mod(psi_e + pi, 2*pi) - pi;
    
    % Calculate lateral position error
    sc2_e = (s(2) - s_ref(2)) * cos(psi_ref) - (s(1) - s_ref(1)) * sin(psi_ref);
    
    % Adjust reference velocity for calculation
    v_e = 0.1;
    if v_ref > v_e || v_ref < -v_e
        v_ref = v_ref;
    elseif v_ref >= 0 && v_ref <= v_e
        v_ref = v_e;
    elseif v_ref >= -v_e && v_ref < 0
        v_ref = -v_e;
    end
    
    % Calculate steering angle error
    delta_e = -(P_p_l / (P_p_Tw^2 * v_ref^2)) * sc2_e - (2 * P_p_l / (P_p_Tw * v_ref)) * psi_e;
end

== matlab function s9_template/Control Software/Position Control/Feed-Forward Control/Create Trajectory  ==
  data: vmax input; u_vp1_t output; xs input; y input; w_p output; t input; P_p_k parameter; P_p_T parameter; P_p_Tt parameter; P_p_kr parameter; P_p_Ti parameter
function [u_vp1_t, w_p] = fcn(vmax, xs, y, t, P_p_k, P_p_T, P_p_Tt, P_p_kr, P_p_Ti)
    % Function: fcn
    % Description: Calculates control signals based on predefined reference polynomials
    %              and time-varying parameters.
    %
    % Inputs:
    %   vmax - Maximum velocity.
    %   xs - Target state variable.
    %   y - Initial state variable.
    %   t - Current time.
    %   P_p_k, P_p_T, P_p_Tt - Parameters for the control dynamics.
    %   P_kr, P_Ti - Parameters for the reference polynomial dynamics.
    %
    % Outputs:
    %   u_vp1_t - Control signal at time t.
    %   w_p - Reference polynomial value at time t.
    %
    % The function computes control signals based on a reference polynomial that is defined 
    % initially and a feedforward polynomial. It uses persistent variables to store the 
    % polynomial coefficients and evaluates them based on the current time 't'. This is useful 
    % for dynamic control systems where the control signal needs to adapt over time.
    
    % Initialize persistent variables if they are empty
    persistent c x0 te cff;
    if isempty(c)
        x0 = y;
        [c, te] = cd_refpoly_vmax(vmax, x0, xs);
        cff = cd_refpoly_ff(c, P_p_k, P_p_T, P_p_Tt, P_p_kr, P_p_Ti);
    end
    
    % Calculate the control signal and reference polynomial value based on current time
    if t >= te
        w_p = polyval(c, te);
        u_vp1_t = polyval(cff, te);
    else
        w_p = polyval(c, t);
        u_vp1_t = polyval(cff, t);
    end
end

== matlab function s9_template/Control Software/v_max switch ==
  data: pos_vmax input; v_ref output; v_max input; type input
function v_ref = fcn(pos_vmax, v_max, type)
    if type == 1
        v_ref = pos_vmax;
    else
        v_ref = v_max;
    end
end

== matlab function s9_template/Control Software/Safety Halt ==
  data: cmd_old input; cmd output; carid input; caroutputsext input; CarInputsCmdHalt parameter; a1total parameter; a2total parameter
function cmd = safety_halt(cmd_old, carid, caroutputsext, CarInputsCmdHalt, a1total, a2total)
    % Function: safety_halt
    % Description: Determines the command for a vehicle to ensure safety, primarily deciding 
    %              whether to continue with the old command or to halt the vehicle.
    %
    % Inputs:
    %   cmd_old - The previous command issued to the vehicle.
    %   carid - Identifier for the specific car.
    %   caroutputsext - Structure containing various car outputs like position, velocity, etc.
    %   CarInputsCmdHalt - Command to halt the vehicle.
    %   a1total - Threshold for the s1 coordinate.
    %   a2total - Threshold for the s2 coordinate.
    %
    % Output:
    %   cmd - The new command for the vehicle, either continuing as before or halting.
    %
    % The function first checks if the car's data is available and valid. If not, or if the car's
    % s1 or s2 coordinates are near the specified thresholds, it issues a halt command. Otherwise,
    % it maintains the previous command.
    %
 
    % % Initial check for data validity and basic conditions
    % if (carid ~= 0) || isempty(caroutputsext.s1) || isempty(caroutputsext.s2) || ...
    %    isempty(caroutputsext.psi) || isempty(caroutputsext.beta) || ...
    %    isempty(caroutputsext.x) || isempty(caroutputsext.v) || ...
    %    isempty(caroutputsext.time)
    %     cmd = CarInputsCmdHalt;
    % else
    %     cmd = cmd_old;
    % end
    % 
    % % Additional check based on position thresholds
    % if caroutputsext.s1 > (a1total - 0.05) || caroutputsext.s2 > (a2total - 0.05) || ...
    %    caroutputsext.s1 < (0 + 0.05) || caroutputsext.s2 < (0 + 0.05)
    %     cmd = CarInputsCmdHalt;
    % else
    %     cmd = cmd_old;
    % end
    cmd = cmd_old;
end

== matlab function s9_template/Vehicle Dynamics/Decision logic u_n ==
  data: u_cmd input; u_n input; u_n output; CarInputsCmdHalt parameter; CarInputsCmdForward parameter; CarInputsCmdReverse parameter
function u_n = fcn(u_cmd, u_n, CarInputsCmdHalt, CarInputsCmdForward, CarInputsCmdReverse)
    % Function: fcn
    % Description: Adjusts the motor control signal based on the current command and
    %              the car's current motor signal state.
    %
    % Inputs:
    %   u_cmd - Current command to the car, dictating its intended movement or action.
    %   u_n - Current motor control signal of the car.
    %   CarInputsCmdHalt - Command value representing the 'Halt' action.
    %   CarInputsCmdForward - Command value representing the 'Move Forward' action.
    %   CarInputsCmdReverse - Command value representing the 'Move Reverse' action.
    %
    % Output:
    %   u_n - Updated motor control signal after applying the command logic.
    %
    % The function updates the motor control signal based on the received command. If the command
    % is to halt, it sets the motor signal to zero. For forward or reverse commands, it adjusts
    % the motor signal appropriately, ensuring no reverse action if moving forward, and vice versa.
    % It also limits the motor signal to a maximum and minimum range.
   
    % Logic to determine the new motor control signal based on the command
    if (u_cmd == CarInputsCmdHalt)
        u_n = 0;
    elseif (u_cmd == CarInputsCmdForward && u_n < 0)
        u_n = 0;
    elseif (u_cmd == CarInputsCmdReverse && u_n > 0)
        u_n = 0;
    elseif u_cmd == CarInputsCmdForward && u_n > 1
        u_n = 1;
    elseif u_cmd == CarInputsCmdReverse && u_n < -1
        u_n = -1;
    else
        u_n = u_n;
    end
end

== matlab function s9_template/Vehicle Dynamics/Conversion to Cartesian coordinates ==
  data: s1_input input; y1 output; s2_input input; psi input; y2 output; P_p_lr parameter
function [y1, y2] = fcn(s1_input, s2_input, psi, P_p_lr)
    % Function: fcn
    % Description: Computes Cartesian coordinates by adjusting input coordinates
    %              with trigonometric transformations.
    %
    % Inputs:
    %   s1_input - Initial x-coordinate or a similar parameter.
    %   s2_input - Initial y-coordinate or a similar parameter.
    %   psi      - Angle in radians, used in the trigonometric transformations.
    %   P_p_lr   - A distance or offset parameter influencing the calculation.
    %
    % Outputs:
    %   y1 - The computed x-coordinate after applying the cosine transformation.
    %   y2 - The computed y-coordinate after applying the sine transformation.
    %
    % The function calculates new Cartesian coordinates (y1, y2) by subtracting
    % the product of P_p_lr and the cosine (for y1) or sine (for y2) of the angle psi
    % from the input coordinates (s1_input, s2_input).
    
    % Calculation of the Cartesian coordinates
    y1 = s1_input - (P_p_lr * cos(psi));
    y2 = s2_input - (P_p_lr * sin(psi));
end

== matlab function s9_template/Vehicle Dynamics/Vehicle Dynamics - HighSpeed/calculate alpha_r ==
  data: v_c1 input; alpha_r output; v_c2 input; psi_p input; P_p_lr parameter
function alpha_r = fcn(v_c1, v_c2, psi_p, P_p_lr)
    % Function: fcn
    % Description: Calculates the rear slip angle 'alpha_r' based on vehicle velocities
    %              and dynamics.
    %
    % Inputs:
    %   v_c1 - Longitudinal component of the center of gravity (COG) velocity.
    %   v_c2 - Lateral component of the COG velocity.
    %   psi_p - Yaw rate of the vehicle.
    %   P_p_lr - Distance from the COG to the rear axle.
    %
    % Output:
    %   alpha_r - Calculated rear slip angle considering the vehicle's dynamics.
    %
    % The function computes the rear slip angle 'alpha_r', taking into account the longitudinal 
    % and lateral velocities of the vehicle's COG, its yaw rate, and the distance from the COG 
    % to the rear axle. The calculation adjusts based on whether the longitudinal velocity 
    % component (v_c1) is positive, negative, or zero.
    
    % Calculation of the rear slip angle 'alpha_r'
    if (v_c1 > 0)
        alpha_r = -atan((v_c2 - (P_p_lr * psi_p)) / v_c1);
    elseif (v_c1 < 0)
        alpha_r = atan((v_c2 - (P_p_lr * psi_p)) / v_c1);
    else 
        alpha_r = 0;
    end
end

== matlab function s9_template/Vehicle Dynamics/Vehicle Dynamics - HighSpeed/Calculate alpha_f ==
  data: v_c1 input; alpha_f output; v_c2 input; psi_p input; delta input; P_p_lf parameter
function alpha_f = fcn(v_c1, v_c2, psi_p, delta, P_p_lf)
    % Function: fcn
    % Description: Calculates the angle 'alpha_f' based on vehicle dynamics and geometry.
    %
    % Inputs:
    %   v_c1 - Longitudinal component of the center of gravity (COG) velocity.
    %   v_c2 - Lateral component of the center of gravity (COG) velocity.
    %   psi_p - Yaw rate of the vehicle.
    %   delta - Steering angle.
    %   P_p_lf - Distance from the COG to the front axle.
    %
    % Output:
    %   alpha_f - Calculated angle factoring in vehicle dynamics and geometry.
    %
    % The function computes the angle 'alpha_f' considering the longitudinal and lateral 
    % components of the COG velocity, the vehicle's yaw rate, and steering angle. It takes 
    % into account the distance from the COG to the rear axle. The computation adjusts 
    % based on whether the longitudinal velocity component (v_c1) is positive, negative, 
    % or zero.

    % Calculation of the angle 'alpha_f'
    if (v_c1 > 0)
        alpha_f = -atan((v_c2 + (P_p_lf * psi_p)) / v_c1) + delta;
    elseif (v_c1 < 0)
        alpha_f = atan((v_c2 + (P_p_lf * psi_p)) / v_c1) - delta;
    else
        alpha_f = 0;
    end
end

== matlab function s9_template/Vehicle Dynamics/Vehicle Dynamics - HighSpeed/Calculate F_f and F_r ==
  data: F_f output; alpha_f input; alpha_r input; F_r output; P_p_Bf parameter; P_p_Cf parameter; P_p_Df parameter; P_p_Ef parameter; P_p_Br parameter; P_p_Cr parameter; P_p_Dr parameter; P_p_Er parameter
function [F_f, F_r] = fcn(alpha_f, alpha_r, P_p_Bf, P_p_Cf, P_p_Df, P_p_Ef, P_p_Br, P_p_Cr, P_p_Dr, P_p_Er)
    % Function: fcn
    % Description: Calculates the tire forces at the front (F_f) and rear (F_r) of the vehicle
    %              using the Magic Formula tire model.
    %
    % Inputs:
    %   alpha_f - Front slip angle.
    %   alpha_r - Rear slip angle.
    %   P_p_Bf, P_p_Cf, P_p_Df, P_p_Ef - Magic Formula coefficients for the front tire.
    %   P_p_Br, P_p_Cr, P_p_Dr, P_p_Er - Magic Formula coefficients for the rear tire.
    %
    % Outputs:
    %   F_f - Calculated tire force at the front.
    %   F_r - Calculated tire force at the rear.
    %
    % The function employs the Magic Formula to compute the tire forces at the front and rear
    % of the vehicle. These forces are crucial for analyzing vehicle dynamics, especially in
    % terms of handling and stability.

    % Calculation of the front and rear tire forces
    F_f = P_p_Df * sin(P_p_Cf * atan(P_p_Bf * (1 - P_p_Ef) * alpha_f - (P_p_Ef * atan(P_p_Bf * alpha_f))));
    F_r = P_p_Dr * sin(P_p_Cr * atan(P_p_Br * (1 - P_p_Er) * alpha_r - (P_p_Er * atan(P_p_Br * alpha_r))));
end

== matlab function s9_template/Vehicle Dynamics/Vehicle Dynamics - HighSpeed/calculate beta ==
  data: v_c1 input; beta output; v_c2 input
function beta = fcn(v_c1, v_c2)
    % Function: fcn
    % Description: Calculates the sideslip angle 'beta' of a vehicle based on its
    %              longitudinal and lateral velocity components.
    %
    % Inputs:
    %   v_c1 - Longitudinal velocity component of the vehicle.
    %   v_c2 - Lateral velocity component of the vehicle.
    %
    % Output:
    %   beta - Calculated sideslip angle.
    %
    % The function uses the 'atan2' function for a more accurate calculation of the
    % angle, especially in cases where the longitudinal velocity component (v_c1) is zero.
    % The sideslip angle 'beta' is an important parameter in vehicle dynamics, representing
    % the angle between the vehicle's direction of motion and the direction it's pointing.
    %
    % Calculation of the sideslip angle 'beta'
    beta = atan2(v_c2, v_c1);
end

== matlab function s9_template/Vehicle Dynamics/Vehicle Dynamics - HighSpeed/calculate s1_p and s2_p ==
  data: v_c1 input; s1_p output; v_c2 input; psi input; s2_p output
function [s1_p, s2_p] = fcn(v_c1, v_c2, psi)
    % Function: fcn
    % Description: Transforms the velocity components from the vehicle's coordinate
    %              system to the global coordinate system.
    %
    % Inputs:
    %   v_c1 - Longitudinal velocity component in the vehicle's coordinate system.
    %   v_c2 - Lateral velocity component in the vehicle's coordinate system.
    %   psi - Yaw angle of the vehicle.
    %
    % Outputs:
    %   s1_p - Transformed longitudinal velocity component in the global coordinate system.
    %   s2_p - Transformed lateral velocity component in the global coordinate system.
    %
    % The function applies a 2D rotation transformation to the velocity components (v_c1, v_c2)
    % based on the vehicle's yaw angle (psi). This transformation is useful for converting
    % vehicle-relative velocities to a global reference frame.

    % Calculating the transformed velocity components
    s1_p = v_c1 * cos(psi) - v_c2 * sin(psi);
    s2_p = v_c1 * sin(psi) + v_c2 * cos(psi);
end
